simulink model "sampleModel358"  (R2021b)
settings: Solver=VariableStepAuto  StartTime=0.0  StopTime=10.0  RelTol=1e-3
undefined symbols (not defined in the file or in its folder): DiscIntNeverNeededParam
libraries: simulink x5
settings Model: Creator=user  LastModifiedBy=user

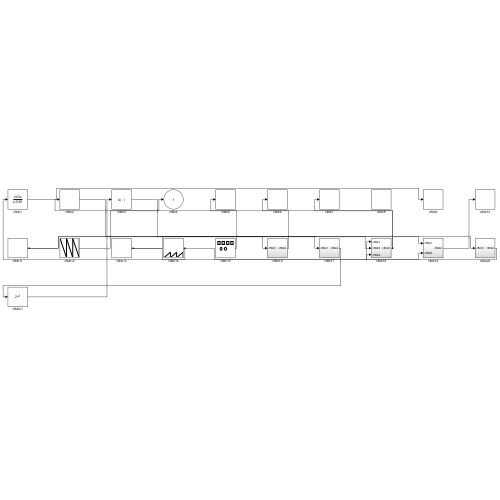
[thumbnail: Simulink's stored preview of the top-level diagram]
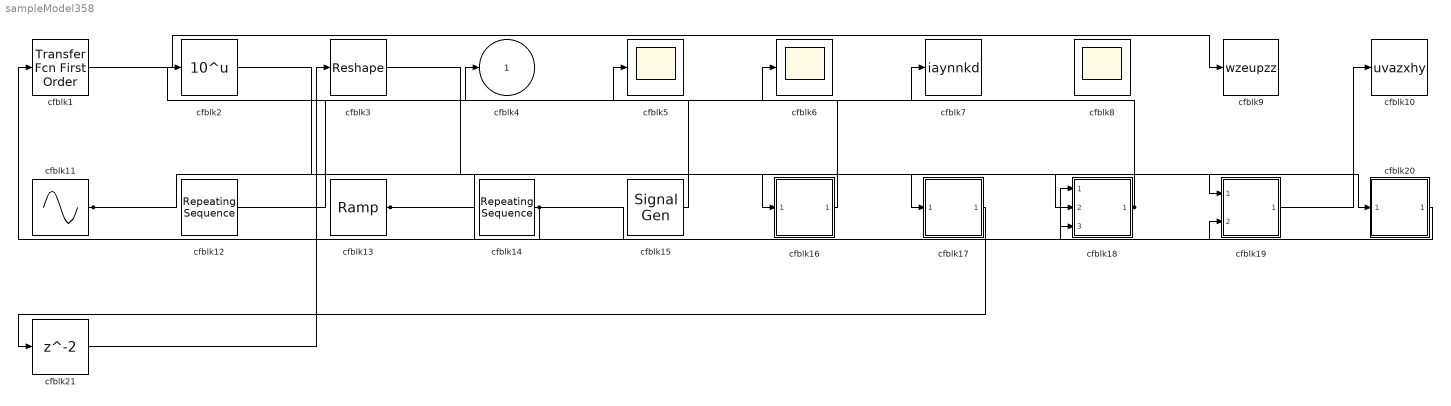
== system sampleModel358 ==
  cfblk1 : simulink/Discrete/Transfer Fcn First Order  PoleZ=0.95  ICPrevOutput=0.0  DoSatur=off
  cfblk10 : ToWorkspace  VariableName=uvazxhy  SaveFormat=Timeseries  SampleTime=-1
  cfblk11 : Sin  Amplitude=[200944024.626752]  Bias=[169774083.790876]  SampleTime=0
  cfblk12 : simulink/Sources/Repeating Sequence  rep_seq_t=[0 2]  rep_seq_y=[536926976.346325, 134798395.358843]
  cfblk13 : simulink/Sources/Ramp  slope=[2287.200617]  start=[27.028139]  InitialOutput=[94605.519158]
  cfblk14 : simulink/Sources/Repeating Sequence  rep_seq_t=[0 2]  rep_seq_y=[-256728306.783110, -183260334.443580]
  cfblk15 : SignalGenerator  Amplitude=[700624424.036884]  Units=rad/sec
  cfblk16 : Subsystem
  cfblk17 : Subsystem
  cfblk18 : Subsystem
  cfblk19 : Subsystem
  cfblk2 : Math  Operator=10^u  SaturateOnIntegerOverflow=on
  cfblk20 : Subsystem
  cfblk21 : Delay  SampleTime=1
  cfblk3 : Reshape
  cfblk5 : Scope
  cfblk6 : Scope
  cfblk7 : ToWorkspace  VariableName=iaynnkd  SaveFormat=Timeseries  SampleTime=-1
  cfblk8 : Scope
      settings: Floating=on
  cfblk9 : ToWorkspace  VariableName=wzeupzz  SaveFormat=Timeseries  SampleTime=-1
  cfblk4 : Outport
  wires:
  cfblk13/1 -> cfblk16/1(cfblk1), cfblk19/2(cfblk4)
  cfblk14/1 -> cfblk1/1, cfblk18/3(cfblk4)
  cfblk1/1 -> cfblk9/1
  cfblk16/1(cfblk2) -> cfblk5/1
  cfblk12/1 -> cfblk4/1
  cfblk3/1 -> cfblk17/1(cfblk1)
  cfblk2/1 -> cfblk19/1(cfblk1)
  cfblk20/1(cfblk2) -> cfblk18/1(cfblk1)
  cfblk18/1(cfblk2) -> cfblk7/1, cfblk6/1
  cfblk11/1 -> cfblk20/1(cfblk1), cfblk18/2(cfblk3)
  cfblk19/1(cfblk2) -> cfblk10/1
  cfblk15/1 -> cfblk2/1
  cfblk17/1(cfblk2) -> cfblk21/1
  cfblk21/1 -> cfblk3/1

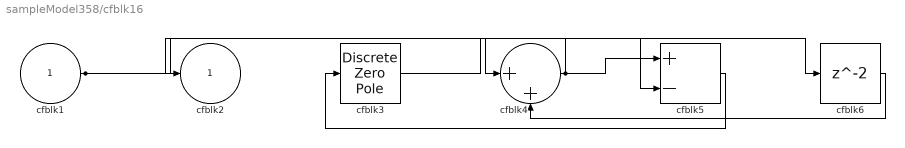
== system sampleModel358/cfblk16 ==
  cfblk1 : Inport
  cfblk3 : DiscreteZeroPole  Poles=[0 0.5]  Gain=1
  cfblk4 : Sum  Inputs=|++
  cfblk5 : Sum  Inputs=+-
  cfblk6 : Delay  SampleTime=1
  cfblk2 : Outport
  wires:
  cfblk1/1 -> cfblk4/1, cfblk5/2
  cfblk4/1 -> cfblk5/1, cfblk2/1
  cfblk5/1 -> cfblk3/1
  cfblk3/1 -> cfblk6/1
  cfblk6/1 -> cfblk4/2

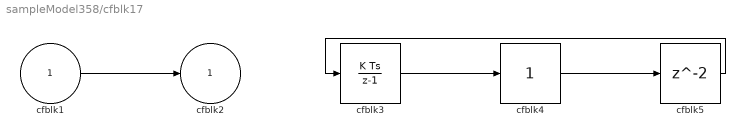
== system sampleModel358/cfblk17 ==
  cfblk1 : Inport
  cfblk3 : DiscreteIntegrator  ICPrevOutput=DiscIntNeverNeededParam  ICPrevScaledInput=DiscIntNeverNeededParam
  cfblk4 : simulink/Math Operations/Slider Gain  gain=1  low=0  high=2
  cfblk5 : Delay  SampleTime=1
  cfblk2 : Outport
  wires:
  cfblk3/1 -> cfblk4/1
  cfblk1/1 -> cfblk2/1
  cfblk4/1 -> cfblk5/1
  cfblk5/1 -> cfblk3/1

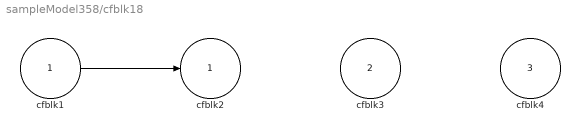
== system sampleModel358/cfblk18 ==
  cfblk1 : Inport
  cfblk3 : Inport  Port=2
  cfblk4 : Inport  Port=3
  cfblk2 : Outport
  wires:
  cfblk1/1 -> cfblk2/1

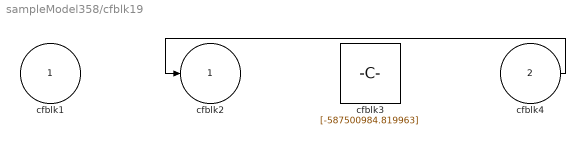
== system sampleModel358/cfblk19 ==
  cfblk1 : Inport
  cfblk4 : Inport  Port=2
  cfblk3 : Constant  Value=[-587500984.819963]  SampleTime=1
  cfblk2 : Outport
  wires:
  cfblk4/1 -> cfblk2/1

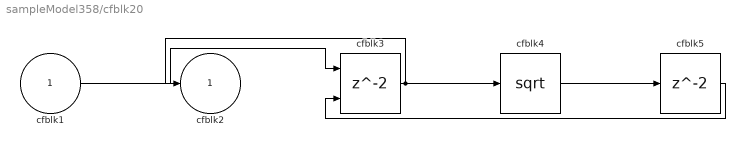
== system sampleModel358/cfblk20 ==
  cfblk1 : Inport
  cfblk3 : Delay  ShowEnablePort=on  SampleTime=1
      settings: InputPortMap=u0,e6
  cfblk4 : Sqrt  SaturateOnIntegerOverflow=on
  cfblk5 : Delay  SampleTime=1
  cfblk2 : Outport
  wires:
  cfblk1/1 -> cfblk3/1
  cfblk3/1 -> cfblk2/1, cfblk4/1
  cfblk4/1 -> cfblk5/1
  cfblk5/1 -> cfblk3/2
